simulink model "Main"  (R2018a)
settings: Solver=VariableStepAuto  StartTime=0.0  StopTime=10  RelTol=1e-3
values from neighbouring files (symbols this model uses):
  A = [0 0 0 0 0 0 0 0 1 0 0 0 0 0 0 0, ... (first row only)    [LQR_G.m]    (also in pole_plasment.m = [)
  B = [0 0 0 0, ... (first row only)    [LQR_G.m]    (also in pole_plasment.m = [)
  C = [1 0 0 0 0 0 0 0 0 0 0 0 0 0 0 0, ... (first row only)    [LQR_G.m]    (also in pole_plasment.m = [)
  K = lqr(A,B,Q,R)    [LQR_G.m]    (also in pole_plasment.m = place(A,B,P))
settings Model: Creator=hussein  LastModifiedBy=hussein
settings DataIOCC: LimitDataPoints=on  SaveOutput=off  SaveTime=off
settings OptimizationCC: BlockReduction=off  BooleanDataType=off  LifeSpan=inf
settings DebuggingCC: SaveWithParameterizedLinksMsg=none  UnderspecifiedInitializationDetection=Classic  MergeDetectMultiDrivingBlocksExec=none  SignalResolutionControl=TryResolveAllWithWarning  AllowSymbolicDim=off  SFUnexpectedBacktrackingDiag=warning  SFNoUnconditionalDefaultTransitionDiag=warning  SFExecutionAtInitializationDiag=none
settings HardwareCC: TargetUnknown=on
settings CodeAppCC: StateflowObjectComments=on
settings GRTTargetCC: TargetLangStandard=C89/C90 (ANSI)  GeneratePreprocessorConditionals=Disable all
settings ConfigComp: CovMetricSettings=dw  CovHtmlReporting=on  CovSaveCumulativeToWorkspaceVar=on  CovSaveSingleToWorkspaceVar=on  CovExternalEMLEnable=off

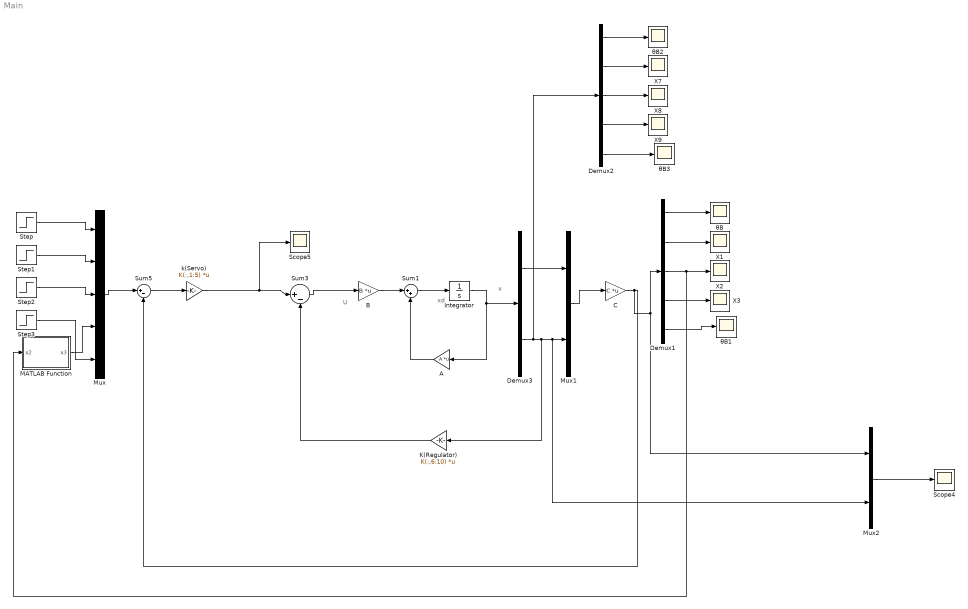
== system Main ==
  note: U
  note: xd
  note: x
  A : Gain  Gain=A  Multiplication=Matrix(K*u)
  B : Gain  Gain=B  Multiplication=Matrix(K*u)
  C : Gain  Gain=C  Multiplication=Matrix(K*u)
  Demux1 : Demux  Outputs=5
  Demux2 : Demux  Outputs=5
  Demux3 : Demux  Outputs=2
  Integrator : Integrator
  K(Regulator) : Gain  Gain=K(:,6:10)  Multiplication=Matrix(K*u)
  MATLAB Function : MATLAB Function  TreatAsAtomicUnit=on
  Mux : Mux  Inputs=5
  Mux1 : Mux  Inputs=2
  Mux2 : Mux  Inputs=2
  Scope4 : Scope
  Scope5 : Scope
  Step : Step  Time=0  SampleTime=0
  Step1 : Step  Time=0  SampleTime=0
  Step2 : Step  Time=0  SampleTime=0
  Step3 : Step  Time=2  After=0  SampleTime=2.1
  Sum1 : Sum  Inputs=|++
  Sum3 : Sum  Inputs=|+-
  Sum5 : Sum  Inputs=|+-
  X{1..3,7..9} (6 alike) : Scope
  k(Servo) : Gain  Gain=K(:,1:5)  Multiplication=Matrix(K*u)
  θB{,1..3} (4 alike) : Scope
  wires:
  B/1 -> Sum1/1
  Sum1/1 -> Integrator/1
  Step/1 -> Mux/1
  Step1/1 -> Mux/2
  Demux1/1 -> θB/1
  Demux1/4 -> X3/1
  Demux1/3 -> MATLAB Function/1(x2), X2/1
  Demux1/2 -> X1/1
  Sum3/1 -> B/1
  Integrator/1 -> A/1, Demux3/1
  A/1 -> Sum1/2
  Mux1/1 -> C/1
  Demux3/1 -> Mux1/1
  Mux/1 -> Sum5/1
  Sum5/1 -> k(Servo)/1
  k(Servo)/1 -> Scope5/1, Sum3/1
  Step2/1 -> Mux/3
  Demux1/5 -> θB1/1
  Demux2/5 -> θB3/1
  Demux2/1 -> θB2/1
  Demux2/4 -> X9/1
  Demux2/2 -> X7/1
  Demux2/3 -> X8/1
  Mux2/1 -> Scope4/1
  C/1 -> Mux2/1, Demux1/1, Sum5/2
  MATLAB Function/1(x3) -> Mux/4
  K(Regulator)/1 -> Sum3/2
  Step3/1 -> Mux/5
  Demux3/2 -> Demux2/1, K(Regulator)/1, Mux2/2, Mux1/2

== matlab function Main/MATLAB Function ==
  data: x2 input; x3 output
function x3 = fcn(x2)
%#codegen
ML=1.73;
x3=((ML+0.23)*x2+9.6*0.25+0.03*0.15)/8.6
